simulink model "test1"  (R2015a)
settings: Solver=ode45  StartTime=0.0  StopTime=50.0  RelTol=1e-3
libraries: simulink x3
settings Model: Creator=dell  LastModifiedBy=dell

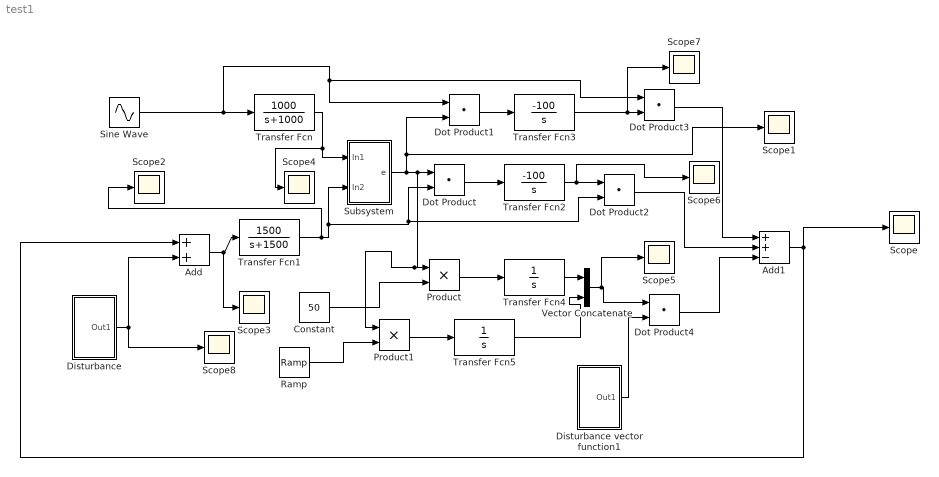
== system test1 ==
  Add : Sum
  Add1 : Sum  Inputs=++-
  Constant : Constant  Value=50
  "Disturbance " : Subsystem
  Disturbance vector function1 : Subsystem
  Dot Product{,1..4} (5 alike) : DotProduct  InputSameDT=on  OutDataTypeStr=Inherit: Inherit via internal rule
  Product : Product
  Product1 : Product
  Ramp : simulink/Sources/Ramp  slope=100  start=0  X0=0
  Scope{,1..8} (9 alike) : Scope
      Scope settings: YMin=-30  YMax=0
      Scope1 settings: YMin=-0.0075  YMax=0.0075
      Scope2 settings: YMin=-1.25  YMax=1.75  SaveName=ScopeData2
      Scope3 settings: SaveName=ScopeData3
      Scope4 settings: TimeRange=0.6890039608875966  YMin=-1  YMax=-0.2  SaveName=ScopeData4
      Scope5 settings: YMin=0.4  YMax=1.3  SaveName=ScopeData5
      Scope6 settings: YMin=-1.5525  YMax=-1.535  SaveName=ScopeData6
      Scope7 settings: YMin=0.255  YMax=0.2615  SaveName=ScopeData7
      Scope8 settings: YMin=2  YMax=2.02  SaveName=ScopeData8
  Sine Wave : Sin  SampleTime=0
  Subsystem : Subsystem
  Transfer Fcn : TransferFcn  Numerator=[1000]  Denominator=[1 1000]
  Transfer Fcn1 : TransferFcn  Numerator=[1500]  Denominator=[1 1500]
  Transfer Fcn2 : TransferFcn  Numerator=[-100]  Denominator=[1 0]
  Transfer Fcn3 : TransferFcn  Numerator=[-100]  Denominator=[1 0]
  Transfer Fcn4 : TransferFcn  Denominator=[1 0]
  Transfer Fcn5 : TransferFcn  Denominator=[1 0]
  Vector Concatenate : Concatenate
  wires:
  Sine Wave/1 -> Dot Product1/1, Dot Product3/1, Transfer Fcn/1
  Add/1 -> Scope3/1, Transfer Fcn1/1
  "Disturbance "/1(Out1) -> Add/2, Scope8/1
  Transfer Fcn/1 -> Scope4/1, Subsystem/1(In1)
  Transfer Fcn1/1 -> Scope2/1, Dot Product2/2, Dot Product/2, Subsystem/2(In2)
  Subsystem/1("e ") -> Product1/1, Product/1, Dot Product/1, Scope1/1, Dot Product1/2
  Dot Product/1 -> Transfer Fcn2/1
  Dot Product1/1 -> Transfer Fcn3/1
  Product/1 -> Transfer Fcn4/1
  Transfer Fcn2/1 -> Scope6/1, Dot Product2/1
  Transfer Fcn3/1 -> Scope7/1, Dot Product3/2
  Vector Concatenate/1 -> Scope5/1, Dot Product4/1
  Disturbance vector function1/1(Out1) -> Dot Product4/2
  Dot Product3/1 -> Add1/1
  Dot Product2/1 -> Add1/2
  Dot Product4/1 -> Add1/3
  Add1/1 -> Add/1, Scope/1
  Ramp/1 -> Product1/2
  Constant/1 -> Product/2
  Product1/1 -> Transfer Fcn5/1
  Transfer Fcn4/1 -> Vector Concatenate/1
  Transfer Fcn5/1 -> Vector Concatenate/2

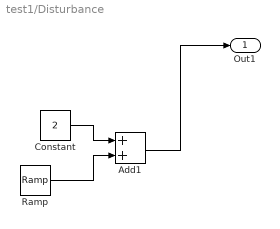
== system test1/Disturbance  ==
  Add1 : Sum
  Constant : Constant  Value=2
  Ramp : simulink/Sources/Ramp  slope=0.5  start=0  X0=0
  Out1 : Outport
  wires:
  Add1/1 -> Out1/1
  Ramp/1 -> Add1/2
  Constant/1 -> Add1/1

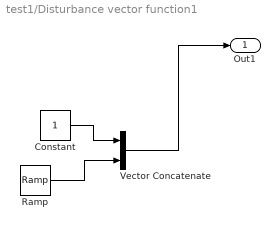
== system test1/Disturbance vector function1 ==
  Constant : Constant
  Ramp : simulink/Sources/Ramp  slope=1  start=0  X0=0
  Vector Concatenate : Concatenate
  Out1 : Outport
  wires:
  Ramp/1 -> Vector Concatenate/2
  Constant/1 -> Vector Concatenate/1
  Vector Concatenate/1 -> Out1/1

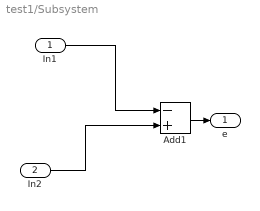
== system test1/Subsystem ==
  In1 : Inport
  In2 : Inport  Port=2
  Add1 : Sum  Inputs=-+
  "e " : Outport
  wires:
  Add1/1 -> "e "/1
  In1/1 -> Add1/1
  In2/1 -> Add1/2
